simulink model "mfordmodel_v1"  (R2023a)
settings: Solver=ode45  StartTime=0.0  StopTime=10.0  RelTol=1e-3  EnableMultiTasking=on
undefined symbols (not defined in the file): ABV_RATIO_SW, AC_OFF_DLY, ACLOD, AUTO_TRNS_SW, BRAKE_DNDT_X, BZZRPM, BZZRPM_ALT, BZZTM, BZZTM_ALT, CMD_LITOFF, CMD_STABLE, CO_ST_ECT__A, COOL_BASE, DAS_BKDLY_A, DAS_CNT, DAS_CTDLY, DAS_LC_SW__A, DASCLP_5INH, DASCTL, DASMHYST, DASMPH, DEBYCP, DES_BASE, DPNEU_MUL, DSDRPM_DN_TC, DSDRPM_OFF, DSDRPM_UP_TC, EDF_DELAY, EDFHP, ETC_CL_TP, ETC_HP, GR_CM_CREEP, HCAM_ACT_CLP, HEDFHP, HEDFRPM, HICAM_PS, IAC_CAL_SW, IAC_ER_TM1, IAC_ER_TM2, IAC_ER_TM4, IAC_HI_LIM__A, IAC_ISFL_OBD, IAC_KAM_SW, IAC_LO_LIM__A, IAC_MON_TM, IAC_OT_REQ, IAC_RUN_TM, IAC_TP_OBD, IAC_TR_DAS, IAC_TST_DC, ID_DAS__A, ID_NOVS__A, IDVS_CH__A, IDVS_SL__A, IPSI_SW, IPSIDLY, IS_DRBASE__A, IS_DRBASE_A__A, IS_NUBASE__A, IS_NUBASE_A__A ... (+35)
libraries: simulink x2
(part 1 of 12)
settings Model: ModifiedHistory=Current Utils Library:utils53_v1.mdl  ExtModeTrigMode=oneshot  Creator=myunt  LastModifiedBy=dkar
settings SolverCC: AlgebraicLoopSolver=TrustRegion
settings DataIOCC: SaveFormat=Array  SignalLoggingSaveFormat=ModelDataLogs  ReturnWorkspaceOutputs=off
settings OptimizationCC: BooleanDataType=off  ExpressionDepthLimit=2147483647  InitFltsAndDblsToZero=on  EfficientMapNaN2IntZero=off  LifeSpan=inf
settings DebuggingCC: SaveWithParameterizedLinksMsg=none  UnderspecifiedInitializationDetection=Classic  MergeDetectMultiDrivingBlocksExec=none  CheckExecutionContextPreStartOutputMsg=on  SignalResolutionControl=TryResolveAllWithWarning  MultiTaskDSMMsg=warning  MultiTaskCondExecSysMsg=none  FcnCallInpInsideContextMsg=warning  UnconnectedInputMsg=warning  UnconnectedOutputMsg=warning  UnconnectedLineMsg=warning  StateNameClashWarn=warning  SFUnexpectedBacktrackingDiag=warning  SFNoUnconditionalDefaultTransitionDiag=warning  SFExecutionAtInitializationDiag=none  ArithmeticOperatorsInVariantConditions=warning
settings HardwareCC: ProdBitPerPointer=32  ProdBitPerSizeT=32  ProdBitPerPtrDiffT=32  ProdLargestAtomicFloat=None  ProdIntDivRoundTo=Undefined  ProdEndianess=Unspecified  ProdWordSize=32  ProdHWDeviceType=32-bit Generic  TargetUnknown=on
settings ModelReferenceCC: PropagateSignalLabelsOutOfModel=off
settings SFSimCC: SimUseLocalCustomCode=off  SimParseCustomCode=off  CustomCodeUndefinedFunction=UseInterfaceOnly
settings RTWCC: RTWUseLocalCustomCode=off
settings CodeAppCC: StateflowObjectComments=on
settings GRTTargetCC: TargetFcnLib=ansi_tfl_tmw.mat  TargetLangStandard=C89/C90 (ANSI)  CombineOutputUpdateFcns=off  GRTInterface=on
settings ConfigComp: CovMetricSettings=dw  CovSaveCumulativeToWorkspaceVar=on  CovSaveSingleToWorkspaceVar=on

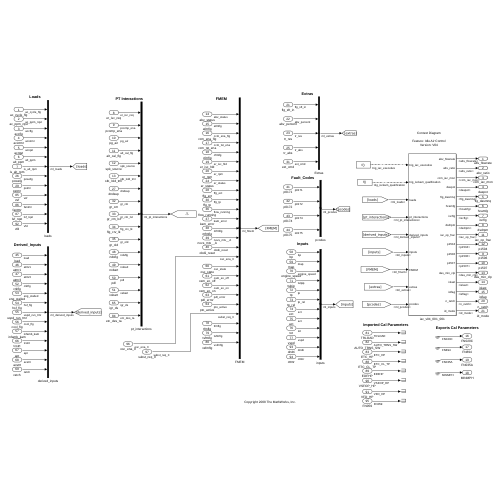
[thumbnail: Simulink's stored preview of the top-level diagram]
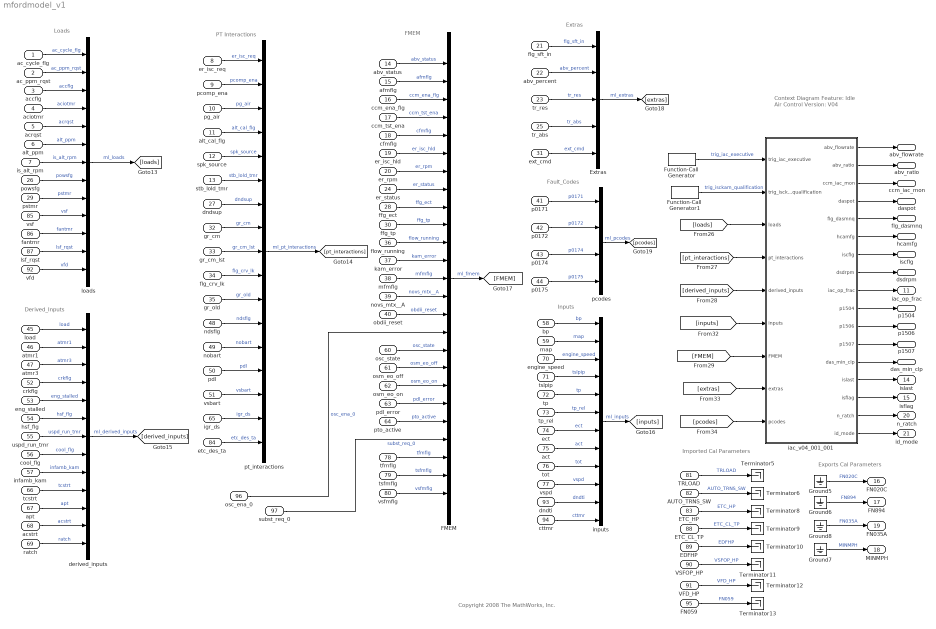
== system mfordmodel_v1 ==
  note: Loads
  note: PT Interactions
  note: Derived_Inputs
  note: Inputs
  note: FMEM
  note: Extras
  note: Context Diagram
      |
      | Feature: Idle Air Control
      | Version: V04
  note: Imported Cal Parameters
  note: Exports Cal Parameters
  note: Fault_Codes
  note: Copyright 2008 The MathWorks, Inc.
  ac_cycle_flg : Inport
  ac_ppm_rqst : Inport  Port=2
  accflg : Inport  Port=3
  aciotmr : Inport  Port=4
  acrqst : Inport  Port=5
  alt_ppm : Inport  Port=6
  is_alt_rpm : Inport  Port=7
  er_isc_req : Inport  Port=8
  pcomp_ena : Inport  Port=9
  pg_air : Inport  Port=10
  alt_cal_flg : Inport  Port=11
  spk_source : Inport  Port=12
  stb_lold_tmr : Inport  Port=13
  abv_status : Inport  Port=14
  afmflg : Inport  Port=15
  ccm_ena_flg : Inport  Port=16
  ccm_tst_ena : Inport  Port=17
  cfmflg : Inport  Port=18
  er_isc_hld : Inport  Port=19
  er_rpm : Inport  Port=20
  flg_sft_in : Inport  Port=21
  abv_percent : Inport  Port=22
  tr_res : Inport  Port=23
  er_status : Inport  Port=24
  tr_abs : Inport  Port=25
  powsfg : Inport  Port=26
  dndsup : Inport  Port=27
  ffg_ect : Inport  Port=28
  pstmr : Inport  Port=29
  ffg_tp : Inport  Port=30
  ext_cmd : Inport  Port=31
  gr_cm : Inport  Port=32
  gr_cm_lst : Inport  Port=33
  flg_crv_lk : Inport  Port=34
  gr_old : Inport  Port=35
  flow_running : Inport  Port=36
  kam_error : Inport  Port=37
  mfmflg : Inport  Port=38
  novs_mtx__A : Inport  Port=39
  obdii_reset : Inport  Port=40
  p0171 : Inport  Port=41
  p0172 : Inport  Port=42
  p0174 : Inport  Port=43
  p0175 : Inport  Port=44
  load : Inport  Port=45
  atmr1 : Inport  Port=46
  atmr3 : Inport  Port=47
  ndsflg : Inport  Port=48
  nobart : Inport  Port=49
  pdl : Inport  Port=50
  vsbart : Inport  Port=51
  crkflg : Inport  Port=52
  eng_stalled : Inport  Port=53
  hsf_flg : Inport  Port=54
  uspd_run_tmr : Inport  Port=55
  cool_flg : Inport  Port=56
  infamb_kam : Inport  Port=57
  bp : Inport  Port=58
  map : Inport  Port=59
  osc_state : Inport  Port=60
  osm_eo_off : Inport  Port=61
  osm_eo_on : Inport  Port=62
  pdl_error : Inport  Port=63
  pto_active : Inport  Port=64
  igr_ds : Inport  Port=65
  tcstrt : Inport  Port=66
  apt : Inport  Port=67
  acstrt : Inport  Port=68
  ratch : Inport  Port=69
  engine_speed : Inport  Port=70
  tslpip : Inport  Port=71
  tp : Inport  Port=72
  tp_rel : Inport  Port=73
  ect : Inport  Port=74
  act : Inport  Port=75
  tot : Inport  Port=76
  vspd : Inport  Port=77
  tfmflg : Inport  Port=78
  tsfmflg : Inport  Port=79
  vsfmflg : Inport  Port=80
  TRLOAD : Inport  Port=81
  AUTO_TRNS_SW : Inport  Port=82
  ETC_HP : Inport  Port=83
  etc_des_ta : Inport  Port=84
  vsf : Inport  Port=85
  fantmr : Inport  Port=86
  lsf_rqst : Inport  Port=87
  ETC_CL_TP : Inport  Port=88
  EDFHP : Inport  Port=89
  VSFOP_HP : Inport  Port=90
  VFD_HP : Inport  Port=91
  vfd : Inport  Port=92
  dndti : Inport  Port=93
  cttmr : Inport  Port=94
  FN059 : Inport  Port=95
  osc_ena_0 : Inport  Port=96
  subst_req_0 : Inport  Port=97
  Extras : Mux  Inputs=5
  FMEM : Mux  Inputs=25
  Function-Call Generator : simulink/Ports & Subsystems/Function-Call Generator  sample_time=0.1  numberOfIterations=1  DisallowWideOutput=off
  Function-Call Generator1 : simulink/Ports & Subsystems/Function-Call Generator  sample_time=0.030  numberOfIterations=1  DisallowWideOutput=off
  Ground{5..8} (4 alike) : Ground
  Terminator{5..6,8..13} (8 alike) : Terminator
  derived_inputs : Mux  Inputs=13
  iac_v04_001_001 : Subsystem
  inputs : Mux  Inputs=12
  loads : Mux  Inputs=13
  pcodes : Mux  Inputs=p0171,p0172,p0174,p0175
  pt_interactions : Mux  Inputs=17
  abv_flowrate : Outport
  abv_ratio : Outport  Port=2
  ccm_iac_mon : Outport  Port=3
  daspot : Outport  Port=4
  flg_dasmnq : Outport  Port=5
  hcamfg : Outport  Port=6
  iscflg : Outport  Port=7
  dsdrpm : Outport  Port=8
  p1506 : Outport  Port=9
  p1507 : Outport  Port=10
  iac_op_frac : Outport  Port=11
  p1504 : Outport  Port=12
  das_min_clp : Outport  Port=13
  islast : Outport  Port=14
  isflag : Outport  Port=15
  FN020C : Outport  Port=16
  FN894 : Outport  Port=17
  MINMPH : Outport  Port=18
  FN035A : Outport  Port=19
  n_ratch : Outport  Port=20
  id_mode : Outport  Port=21
  wires:
  ac_ppm_rqst/1 -> loads/2  "ac_ppm_rqst"
  ac_cycle_flg/1 -> loads/1  "ac_cycle_flg"
  loads/1 -> [loads]  "ml_loads"
  er_isc_req/1 -> pt_interactions/1  "er_isc_req"
  pg_air/1 -> pt_interactions/3  "pg_air"
  pcomp_ena/1 -> pt_interactions/2  "pcomp_ena"
  spk_source/1 -> pt_interactions/5  "spk_source"
  stb_lold_tmr/1 -> pt_interactions/6  "stb_lold_tmr"
  alt_cal_flg/1 -> pt_interactions/4  "alt_cal_flg"
  pt_interactions/1 -> [pt_interactions]  "ml_pt_interactions"
  Extras/1 -> [extras]  "ml_extras"
  accflg/1 -> loads/3  "accflg"
  aciotmr/1 -> loads/4  "aciotmr"
  acrqst/1 -> loads/5  "acrqst"
  is_alt_rpm/1 -> loads/7  "is_alt_rpm"
  alt_ppm/1 -> loads/6  "alt_ppm"
  [pt_interactions] -> iac_v04_001_001/4(pt_interactions)
  [derived_inputs] -> iac_v04_001_001/5(derived_inputs)
  [inputs] -> iac_v04_001_001/6(inputs)
  [extras] -> iac_v04_001_001/8(extras)
  TRLOAD/1 -> Terminator5/1  "TRLOAD"
  AUTO_TRNS_SW/1 -> Terminator6/1  "AUTO_TRNS_SW"
  Ground5/1 -> FN020C/1  "FN020C"
  Ground6/1 -> FN894/1  "FN894"
  [pcodes] -> iac_v04_001_001/9(pcodes)
  Ground7/1 -> MINMPH/1  "MINMPH"
  Ground8/1 -> FN035A/1  "FN035A"
  FMEM/1 -> [FMEM]  "ml_fmem"
  osc_state/1 -> FMEM/17  "osc_state"
  osm_eo_off/1 -> FMEM/18  "osm_eo_off"
  osm_eo_on/1 -> FMEM/19  "osm_eo_on"
  pdl_error/1 -> FMEM/20  "pdl_error"
  pto_active/1 -> FMEM/21  "pto_active"
  tfmflg/1 -> FMEM/23  "tfmflg"
  tsfmflg/1 -> FMEM/24  "tsfmflg"
  derived_inputs/1 -> [derived_inputs]  "ml_derived_inputs"
  load/1 -> derived_inputs/1  "load"
  atmr1/1 -> derived_inputs/2  "atmr1"
  atmr3/1 -> derived_inputs/3  "atmr3"
  crkflg/1 -> derived_inputs/4  "crkflg"
  eng_stalled/1 -> derived_inputs/5  "eng_stalled"
  hsf_flg/1 -> derived_inputs/6  "hsf_flg"
  uspd_run_tmr/1 -> derived_inputs/7  "uspd_run_tmr"
  cool_flg/1 -> derived_inputs/8  "cool_flg"
  infamb_kam/1 -> derived_inputs/9  "infamb_kam"
  tcstrt/1 -> derived_inputs/10  "tcstrt"
  apt/1 -> derived_inputs/11  "apt"
  acstrt/1 -> derived_inputs/12  "acstrt"
  ratch/1 -> derived_inputs/13  "ratch"
  osc_ena_0/1 -> FMEM/16  "osc_ena_0"
  subst_req_0/1 -> FMEM/22  "subst_req_0"
  dndsup/1 -> pt_interactions/7  "dndsup"
  gr_cm/1 -> pt_interactions/8  "gr_cm"
  gr_cm_lst/1 -> pt_interactions/9  "gr_cm_lst"
  flg_crv_lk/1 -> pt_interactions/10  "flg_crv_lk"
  gr_old/1 -> pt_interactions/11  "gr_old"
  ndsflg/1 -> pt_interactions/12  "ndsflg"
  pdl/1 -> pt_interactions/14  "pdl"
  vsbart/1 -> pt_interactions/15  "vsbart"
  igr_ds/1 -> pt_interactions/16  "igr_ds"
  etc_des_ta/1 -> pt_interactions/17  "etc_des_ta"
  nobart/1 -> pt_interactions/13  "nobart"
  powsfg/1 -> loads/8  "powsfg"
  pstmr/1 -> loads/9  "pstmr"
  vsf/1 -> loads/10  "vsf"
  fantmr/1 -> loads/11  "fantmr"
  lsf_rqst/1 -> loads/12  "lsf_rqst"
  vfd/1 -> loads/13  "vfd"
  vsfmflg/1 -> FMEM/25  "vsfmflg"
  abv_status/1 -> FMEM/1  "abv_status"
  afmflg/1 -> FMEM/2  "afmflg"
  ccm_ena_flg/1 -> FMEM/3  "ccm_ena_flg"
  ccm_tst_ena/1 -> FMEM/4  "ccm_tst_ena"
  cfmflg/1 -> FMEM/5  "cfmflg"
  er_isc_hld/1 -> FMEM/6  "er_isc_hld"
  er_status/1 -> FMEM/8  "er_status"
  ffg_ect/1 -> FMEM/9  "ffg_ect"
  ffg_tp/1 -> FMEM/10  "ffg_tp"
  flow_running/1 -> FMEM/11  "flow_running"
  er_rpm/1 -> FMEM/7  "er_rpm"
  kam_error/1 -> FMEM/12  "kam_error"
  mfmflg/1 -> FMEM/13  "mfmflg"
  novs_mtx__A/1 -> FMEM/14  "novs_mtx__A"
  obdii_reset/1 -> FMEM/15  "obdii_reset"
  flg_sft_in/1 -> Extras/1  "flg_sft_in"
  abv_percent/1 -> Extras/2  "abv_percent"
  tr_res/1 -> Extras/3  "tr_res"
  tr_abs/1 -> Extras/4  "tr_abs"
  ext_cmd/1 -> Extras/5  "ext_cmd"
  pcodes/1 -> [pcodes]  "ml_pcodes"
  p0171/1 -> pcodes/1  "p0171"
  p0172/1 -> pcodes/2  "p0172"
  p0174/1 -> pcodes/3  "p0174"
  p0175/1 -> pcodes/4  "p0175"
  ect/1 -> inputs/7  "ect"
  act/1 -> inputs/8  "act"
  tot/1 -> inputs/9  "tot"
  tp/1 -> inputs/5  "tp"
  tp_rel/1 -> inputs/6  "tp_rel"
  tslpip/1 -> inputs/4  "tslpip"
  engine_speed/1 -> inputs/3  "engine_speed"
  map/1 -> inputs/2  "map"
  bp/1 -> inputs/1  "bp"
  vspd/1 -> inputs/10  "vspd"
  inputs/1 -> [inputs]  "ml_inputs"
  dndti/1 -> inputs/11  "dndti"
  cttmr/1 -> inputs/12  "cttmr"
  ETC_HP/1 -> Terminator8/1  "ETC_HP"
  ETC_CL_TP/1 -> Terminator9/1  "ETC_CL_TP"
  EDFHP/1 -> Terminator10/1  "EDFHP"
  VSFOP_HP/1 -> Terminator11/1  "VSFOP_HP"
  VFD_HP/1 -> Terminator12/1  "VFD_HP"
  iac_v04_001_001/3(ccm_iac_mon) -> ccm_iac_mon/1
  iac_v04_001_001/5(flg_dasmnq) -> flg_dasmnq/1
  iac_v04_001_001/12(p1507) -> p1507/1
  iac_v04_001_001/2(abv_ratio) -> abv_ratio/1
  iac_v04_001_001/4(daspot) -> daspot/1
  iac_v04_001_001/6(hcamfg) -> hcamfg/1
  iac_v04_001_001/7(iscflg) -> iscflg/1
  iac_v04_001_001/11(p1506) -> p1506/1
  iac_v04_001_001/1(abv_flowrate) -> abv_flowrate/1
  iac_v04_001_001/8(dsdrpm) -> dsdrpm/1
  iac_v04_001_001/9(iac_op_frac) -> iac_op_frac/1
  iac_v04_001_001/10(p1504) -> p1504/1
  iac_v04_001_001/13(das_min_clp) -> das_min_clp/1
  iac_v04_001_001/14(islast) -> islast/1
  iac_v04_001_001/15(isflag) -> isflag/1
  iac_v04_001_001/16(n_ratch) -> n_ratch/1
  iac_v04_001_001/17(id_mode) -> id_mode/1
  [loads] -> iac_v04_001_001/3(loads)
  [FMEM] -> iac_v04_001_001/7(FMEM)
  Function-Call Generator1/1 -> iac_v04_001_001/2(trig_isckam_qualification)  "trig_isckam_qualification"
  Function-Call Generator/1 -> iac_v04_001_001/1(trig_iac_executive)  "trig_iac_executive"
  FN059/1 -> Terminator13/1  "FN059"

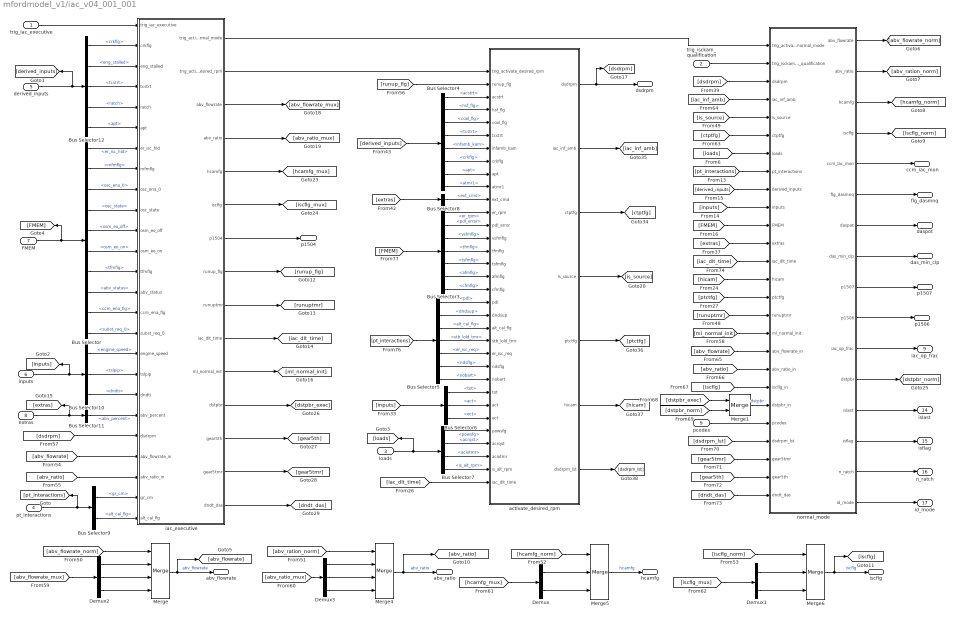
== system mfordmodel_v1/iac_v04_001_001 ==
  trig_iac_executive : Inport
  trig_isckam_qualification : Inport  Port=2
  loads : Inport  Port=3
  pt_interactions : Inport  Port=4
  derived_inputs : Inport  Port=5
  inputs : Inport  Port=6
  FMEM : Inport  Port=7
  extras : Inport  Port=8
  pcodes : Inport  Port=9
  Bus Selector : BusSelector  OutputSignals=er_isc_hld,mfmflg,osc_ena_0,osc_state,osm_eo_off,osm_eo_on,tfmflg,abv_status,ccm_ena_flg,subst_req_0
  Bus Selector10 : BusSelector  OutputSignals=engine_speed,tslpip,dndti
  Bus Selector11 : BusSelector  OutputSignals=abv_percent
  Bus Selector12 : BusSelector  OutputSignals=crkflg,eng_stalled,tcstrt,ratch,apt
  Bus Selector3 : BusSelector  OutputSignals=er_rpm,pdl_error,vsfmflg,tfmflg,tsfmflg,afmflg,cfmflg
  Bus Selector4 : BusSelector  OutputSignals=acstrt,hsf_flg,cool_flg,tcstrt,infamb_kam,crkflg,apt,atmr1
  Bus Selector5 : BusSelector  OutputSignals=pdl,dndsup,alt_cal_flg,stb_lold_tmr,er_isc_req,ndsflg,nobart
  Bus Selector6 : BusSelector  OutputSignals=tot,act,ect
  Bus Selector7 : BusSelector  OutputSignals=powsfg,acrqst,aciotmr,is_alt_rpm
  Bus Selector8 : BusSelector  OutputSignals=ext_cmd
  Bus Selector9 : BusSelector  OutputSignals=gr_cm,alt_cal_flg
  Demux : Demux  Outputs=2
      settings: DisplayOption=none
  Demux1 : Demux  Outputs=2
      settings: DisplayOption=none
  Demux2 : Demux  Outputs=3
      settings: DisplayOption=none
  Demux3 : Demux  Outputs=3
      settings: DisplayOption=none
  Merge : Merge  Inputs=4
  Merge1 : Merge
  Merge4 : Merge  Inputs=4
  Merge5 : Merge  Inputs=3
  Merge6 : Merge  Inputs=3
  activate_desired_rpm : Subsystem
  iac_executive : Subsystem
  normal_mode : Subsystem
  abv_flowrate : Outport
  abv_ratio : Outport  Port=2
  ccm_iac_mon : Outport  Port=3
  daspot : Outport  Port=4
  flg_dasmnq : Outport  Port=5
  hcamfg : Outport  Port=6
  iscflg : Outport  Port=7
  dsdrpm : Outport  Port=8
  iac_op_frac : Outport  Port=9
  p1504 : Outport  Port=10
  p1506 : Outport  Port=11
  p1507 : Outport  Port=12
  das_min_clp : Outport  Port=13
  islast : Outport  Port=14
  isflag : Outport  Port=15
  n_ratch : Outport  Port=16
  id_mode : Outport  Port=17
  wires:
  normal_mode/16(id_mode) -> id_mode/1
  normal_mode/15(n_ratch) -> n_ratch/1
  normal_mode/11(iac_op_frac) -> iac_op_frac/1
  normal_mode/9(p1507) -> p1507/1
  normal_mode/6(flg_dasmnq) -> flg_dasmnq/1
  normal_mode/5(ccm_iac_mon) -> ccm_iac_mon/1
  normal_mode/7(daspot) -> daspot/1
  normal_mode/8(das_min_clp) -> das_min_clp/1
  normal_mode/14(isflag) -> isflag/1
  normal_mode/13(islast) -> islast/1
  normal_mode/10(p1506) -> p1506/1
  Demux1/1 -> Merge6/2
  Demux1/2 -> Merge6/3
  Merge6/1 -> iscflg/1, [iscflg]  "iscflg"
  [iscflg_mux] -> Demux1/1
  [iscflg_norm] -> Merge6/1
  Demux/1 -> Merge5/2
  Demux/2 -> Merge5/3
  Merge5/1 -> hcamfg/1  "hcamfg"
  [hcamfg_mux] -> Demux/1
  Demux2/3 -> Merge/4
  Demux2/1 -> Merge/2
  [abv_flowrate_norm] -> Merge/1
  Merge/1 -> abv_flowrate/1, [abv_flowrate]  "abv_flowrate"
  [abv_flowrate_mux] -> Demux2/1
  Demux2/2 -> Merge/3
  derived_inputs/1 -> Bus Selector12/1, [derived_inputs]
  Bus Selector12/5 -> iac_executive/6(apt)  "<apt>"
  pt_interactions/1 -> Bus Selector9/1, [pt_interactions]
  Bus Selector9/1 -> iac_executive/24(gr_cm)  "<gr_cm>"
  Bus Selector9/2 -> iac_executive/25(alt_cal_flg)  "<alt_cal_flg>"
  extras/1 -> Bus Selector11/1, [extras]
  Bus Selector11/1 -> iac_executive/20(abv_percent)  "<abv_percent>"
  [dsdrpm] -> iac_executive/21(dsdrpm)
  [abv_flowrate] -> iac_executive/22(abv_flowrate_in)
  [abv_ratio] -> iac_executive/23(abv_ratio_in)
  inputs/1 -> Bus Selector10/1, [inputs]
  Bus Selector10/3 -> iac_executive/19(dndti)  "<dndti>"
  Bus Selector10/1 -> iac_executive/17(engine_speed)  "<engine_speed>"
  Bus Selector10/2 -> iac_executive/18(tslpip)  "<tslpip>"
  FMEM/1 -> Bus Selector/1, [FMEM]
  Bus Selector/2 -> iac_executive/8(mfmflg)  "<mfmflg>"
  Bus Selector/3 -> iac_executive/9(osc_ena_0)  "<osc_ena_0>"
  Bus Selector/4 -> iac_executive/10(osc_state)  "<osc_state>"
  Bus Selector/5 -> iac_executive/11(osm_eo_off)  "<osm_eo_off>"
  Bus Selector/6 -> iac_executive/12(osm_eo_on)  "<osm_eo_on>"
  Bus Selector/7 -> iac_executive/13(tfmflg)  "<tfmflg>"
  Bus Selector/8 -> iac_executive/14(abv_status)  "<abv_status>"
  Bus Selector/10 -> iac_executive/16(subst_req_0)  "<subst_req_0>"
  Bus Selector/9 -> iac_executive/15(ccm_ena_flg)  "<ccm_ena_flg>"
  Bus Selector12/1 -> iac_executive/2(crkflg)  "<crkflg>"
  Bus Selector12/2 -> iac_executive/3(eng_stalled)  "<eng_stalled>"
  trig_iac_executive/1 -> iac_executive/1(trig_iac_executive)
  Bus Selector/1 -> iac_executive/7(er_isc_hld)  "<er_isc_hld>"
  Bus Selector12/3 -> iac_executive/4(tcstrt)  "<tcstrt>"
  Bus Selector12/4 -> iac_executive/5(ratch)  "<ratch>"
  iac_executive/7(p1504) -> p1504/1
  Bus Selector5/7 -> activate_desired_rpm/25(nobart)  "<nobart>"
  [dstpbr_exec] -> Merge1/1
  [dstpbr_norm] -> Merge1/2
  [gear5tmr] -> normal_mode/24(gear5tmr)
  [dndt_das] -> normal_mode/26(dndt_das)
  [gear5th] -> normal_mode/25(gear5th)
  pcodes/1 -> normal_mode/22(pcodes)
  iac_executive/15(dndt_das) -> [dndt_das]
  iac_executive/14(gear5tmr) -> [gear5tmr]
  iac_executive/13(gear5th) -> [gear5th]
  [derived_inputs] -> Bus Selector4/1
  Bus Selector8/1 -> activate_desired_rpm/11(ext_cmd)  "<ext_cmd>"
  [extras] -> Bus Selector8/1
  [FMEM] -> Bus Selector3/1
  Bus Selector3/1 -> activate_desired_rpm/12(er_rpm)  "<er_rpm>"
  Bus Selector3/2 -> activate_desired_rpm/13(pdl_error)  "<pdl_error>"
  Bus Selector3/3 -> activate_desired_rpm/14(vsfmflg)  "<vsfmflg>"
  Bus Selector3/4 -> activate_desired_rpm/15(tfmflg)  "<tfmflg>"
  Bus Selector3/5 -> activate_desired_rpm/16(tsfmflg)  "<tsfmflg>"
  Bus Selector3/6 -> activate_desired_rpm/17(afmflg)  "<afmflg>"
  Bus Selector3/7 -> activate_desired_rpm/18(cfmflg)  "<cfmflg>"
  [pt_interactions] -> Bus Selector5/1
  [dsdrpm_lst] -> normal_mode/23(dsdrpm_lst)
  [FMEM] -> normal_mode/11(FMEM)
  [inputs] -> normal_mode/10(inputs)
  [dsdrpm] -> normal_mode/3(dsdrpm)
  [hicam] -> normal_mode/14(hicam)
  [ptctfg] -> normal_mode/15(ptctfg)
  trig_isckam_qualification/1 -> normal_mode/2(trig_isckam_qualification)
  activate_desired_rpm/7(dsdrpm_lst) -> [dsdrpm_lst]
  normal_mode/1(abv_flowrate) -> [abv_flowrate_norm]
  normal_mode/3(hcamfg) -> [hcamfg_norm]
  normal_mode/4(iscflg) -> [iscflg_norm]
  normal_mode/2(abv_ratio) -> [abv_ration_norm]
  Bus Selector7/1 -> activate_desired_rpm/29(powsfg)  "<powsfg>"
  Bus Selector7/2 -> activate_desired_rpm/30(acrqst)  "<acrqst>"
  Bus Selector7/3 -> activate_desired_rpm/31(aciotmr)  "<aciotmr>"
  Bus Selector7/4 -> activate_desired_rpm/32(is_alt_rpm)  "<is_alt_rpm>"
  Bus Selector4/1 -> activate_desired_rpm/3(acstrt)  "<acstrt>"
  Bus Selector4/2 -> activate_desired_rpm/4(hsf_flg)  "<hsf_flg>"
  Bus Selector4/3 -> activate_desired_rpm/5(cool_flg)  "<cool_flg>"
  Bus Selector4/4 -> activate_desired_rpm/6(tcstrt)  "<tcstrt>"
  Bus Selector4/5 -> activate_desired_rpm/7(infamb_kam)  "<infamb_kam>"
  Bus Selector4/6 -> activate_desired_rpm/8(crkflg)  "<crkflg>"
  Bus Selector4/7 -> activate_desired_rpm/9(apt)  "<apt>"
  Bus Selector4/8 -> activate_desired_rpm/10(atmr1)  "<atmr1>"
  Bus Selector5/1 -> activate_desired_rpm/19(pdl)  "<pdl>"
  Bus Selector5/2 -> activate_desired_rpm/20(dndsup)  "<dndsup>"
  Bus Selector5/3 -> activate_desired_rpm/21(alt_cal_flg)  "<alt_cal_flg>"
  Bus Selector5/4 -> activate_desired_rpm/22(stb_lold_tmr)  "<stb_lold_tmr>"
  Bus Selector5/5 -> activate_desired_rpm/23(er_isc_req)  "<er_isc_req>"
  Bus Selector5/6 -> activate_desired_rpm/24(ndsflg)  "<ndsflg>"
  [runup_flg] -> activate_desired_rpm/2(runup_flg)
  activate_desired_rpm/2(iac_inf_amb) -> [iac_inf_amb]
  activate_desired_rpm/3(ctptfg) -> [ctptfg]
  activate_desired_rpm/4(is_source) -> [is_source]
  activate_desired_rpm/5(ptctfg) -> [ptctfg]
  [iac_dlt_time] -> activate_desired_rpm/33(iac_dlt_time)
  activate_desired_rpm/6(hicam) -> [hicam]
  Merge1/1 -> normal_mode/21(dstpbr_in)  "dstpbr"
  loads/1 -> Bus Selector7/1, [loads]
  Bus Selector6/1 -> activate_desired_rpm/26(tot)  "<tot>"
  Bus Selector6/2 -> activate_desired_rpm/27(act)  "<act>"
  Bus Selector6/3 -> activate_desired_rpm/28(ect)  "<ect>"
  [inputs] -> Bus Selector6/1
  [hcamfg_norm] -> Merge5/1
  activate_desired_rpm/1(dsdrpm) -> [dsdrpm], dsdrpm/1
  iac_executive/1(trig_activate_normal_mode) -> normal_mode/1(trig_activate_normal_mode)
  iac_executive/8(runup_flg) -> [runup_flg]
  iac_executive/10(iac_dlt_time) -> [iac_dlt_time]
  iac_executive/9(runuptmr) -> [runuptmr]
  iac_executive/2(trig_activate_desired_rpm) -> activate_desired_rpm/1(trig_activate_desired_rpm)
  iac_executive/11(ml_normal_init) -> [ml_normal_init]
  iac_executive/3(abv_flowrate) -> [abv_flowrate_mux]
  iac_executive/4(abv_ratio) -> [abv_ratio_mux]
  iac_executive/5(hcamfg) -> [hcamfg_mux]
  iac_executive/6(iscflg) -> [iscflg_mux]
  iac_executive/12(dstpbr) -> [dstpbr_exec]
  Demux3/3 -> Merge4/4
  [abv_ration_norm] -> Merge4/1
  Demux3/1 -> Merge4/2
  Demux3/2 -> Merge4/3
  Merge4/1 -> abv_ratio/1, [abv_ratio]  "abv_ratio"
  [abv_ratio_mux] -> Demux3/1
  [loads] -> normal_mode/7(loads)
  [pt_interactions] -> normal_mode/8(pt_interactions)
  [derived_inputs] -> normal_mode/9(derived_inputs)
  [extras] -> normal_mode/12(extras)
  [iac_dlt_time] -> normal_mode/13(iac_dlt_time)
  [is_source] -> normal_mode/5(is_source)
  [ctptfg] -> normal_mode/6(ctptfg)
  [iac_inf_amb] -> normal_mode/4(iac_inf_amb)
  [runuptmr] -> normal_mode/16(runuptmr)
  [ml_normal_init] -> normal_mode/17(ml_normal_init)
  [abv_flowrate] -> normal_mode/18(abv_flowrate_in)
  [abv_ratio] -> normal_mode/19(abv_ratio_in)
  [iscflg] -> normal_mode/20(iscflg_in)
  normal_mode/12(dstpbr) -> [dstpbr_norm]

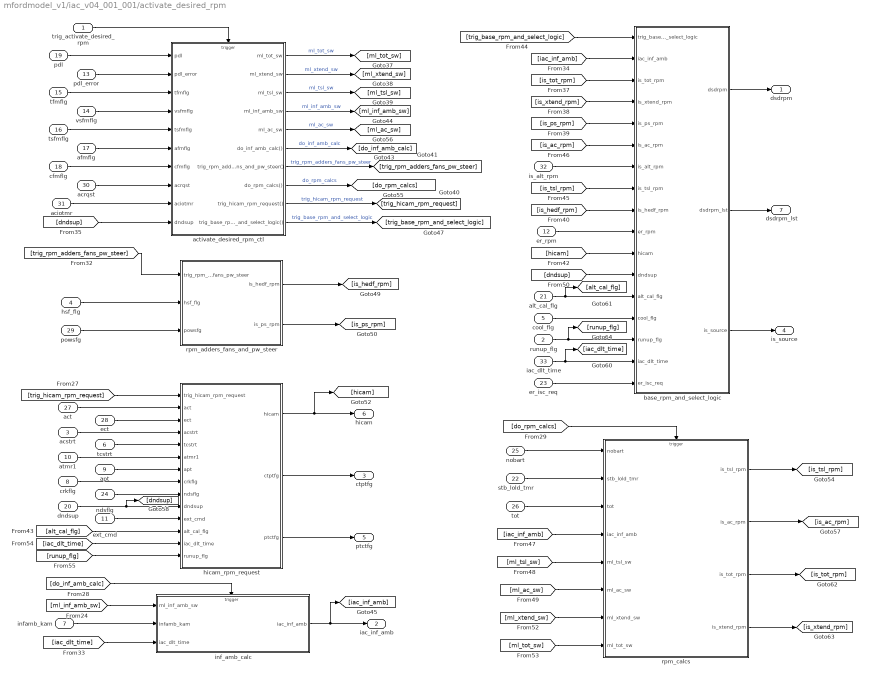
== system mfordmodel_v1/iac_v04_001_001/activate_desired_rpm ==
  trig_activate_desired_rpm : Inport
  runup_flg : Inport  Port=2
  acstrt : Inport  Port=3
  hsf_flg : Inport  Port=4
  cool_flg : Inport  Port=5
  tcstrt : Inport  Port=6
  infamb_kam : Inport  Port=7
  crkflg : Inport  Port=8
  apt : Inport  Port=9
  atmr1 : Inport  Port=10
  ext_cmd : Inport  Port=11
  er_rpm : Inport  Port=12
  pdl_error : Inport  Port=13
  vsfmflg : Inport  Port=14
  tfmflg : Inport  Port=15
  tsfmflg : Inport  Port=16
  afmflg : Inport  Port=17
  cfmflg : Inport  Port=18
  pdl : Inport  Port=19
  dndsup : Inport  Port=20
  alt_cal_flg : Inport  Port=21
  stb_lold_tmr : Inport  Port=22
  er_isc_req : Inport  Port=23
  ndsflg : Inport  Port=24
  nobart : Inport  Port=25
  tot : Inport  Port=26
  act : Inport  Port=27
  ect : Inport  Port=28
  powsfg : Inport  Port=29
  acrqst : Inport  Port=30
  aciotmr : Inport  Port=31
  is_alt_rpm : Inport  Port=32
  iac_dlt_time : Inport  Port=33
  activate_desired_rpm_ctl : Stateflow chart  TreatAsAtomicUnit=on
  base_rpm_and_select_logic : Subsystem
  hicam_rpm_request : Subsystem
  inf_amb_calc : Subsystem  TreatAsAtomicUnit=on  mask(inf_amb_calc){}
      mask help: TBD
      mask Display:
      | disp('
      | IF (ml_inf_amb_sw == 1)  THEN                              \n
      | iac_inf_amb = infamb_kam                              \n
      | ELSE IF (ml_inf_amb_sw == 2) THEN                     \n
      | iac_inf_amb = rolav_tc (iac_inf_amb,              \n
      | 254.0, iac_delta_time, 16)\n
      | ENDIF                                                                      ')
  rpm_adders_fans_and_pw_steer : Subsystem  mask(rpm_adders_fans_and_pw_steer){}
      mask help: Calculate the HEDF and PS RPM requests.
      mask Display:
      | disp('
      | IF ( ( HEDFHP == 1) AND      \n
      | ( HSF_FLG == 1))      \n
      | is_hedf_rpm = HEDFRPM\n
      | ELSE                                       \n
      | is_hedf_rpm = 0                \n
      | ENDIF                                    \n \n
      | IF (powsfg == 1)                     \n
      | is_ps_rpm = PS_RPM      \n
      | ELSE                                      \n
      | is_ps_rpm  = 0                  \n
      | ENDIF                                     ')
  rpm_calcs : Subsystem  TreatAsAtomicUnit=on  mask(rpm_calcs){}
      mask help: TBD
      mask Display:
      | disp('
      | IF (ml_tsl_sw == 1) THEN                          \n
      | is_tsl_rpm = 0.0                                    \n
      | ELSE IF (ml_tsl_sw == 2) THEN                \n
      | is_tsl_rpm = ( nobart * RT_CHAIN        \n
      |  * COAST_FRAC )\n
      | ENDIF                                                         \n\n
      | IF (ml_tot_sw == 1 ) THEN                         \n
      | is_tot_rpm = FN861R(tot)                   \n
      | ELSE IF (ml_tot_sw == 2) THEN                \n
      | is_tot_rpm = FN861(tot)                     \n
      | ENDIF                                                          \n\n
      | IF (ml_ac_sw == 1) THEN                           \n
      | is_ac_rpm = FNIAC_AC_N(iac_inf_amb)\n
      | ELSE IF (ml_ac_sw == 2) THEN                  \n
      | is_ac_rpm = FNIAC_AC_D(iac_inf_amb)\n
      | ELSE IF (ml_ac_sw == 3 THEN                   \n
      | is_ac_rpm = 0.0                                        \n
      | ENDIF                                                           \n\n
      | IF (is_xtend_rpm == 1) THEN                       \n
      | is_xtend_rpm = FN880N(stblold_tmr)     \n
      | ELSE IF (ml_xtend_sw == 2) THEN              \n
      | is_xtend_rpm = 0.0                                  \n
      | ENDIF                                                            ')
  dsdrpm : Outport
  iac_inf_amb : Outport  Port=2
  ctptfg : Outport  Port=3
  is_source : Outport  Port=4
  ptctfg : Outport  Port=5
  hicam : Outport  Port=6
  dsdrpm_lst : Outport  Port=7
  wires:
  vsfmflg/1 -> activate_desired_rpm_ctl/4(vsfmflg)
  alt_cal_flg/1 -> [alt_cal_flg], base_rpm_and_select_logic/13(alt_cal_flg)
  [ml_tot_sw] -> rpm_calcs/8(ml_tot_sw)
  [ml_xtend_sw] -> rpm_calcs/7(ml_xtend_sw)
  [ml_ac_sw] -> rpm_calcs/6(ml_ac_sw)
  [ml_tsl_sw] -> rpm_calcs/5(ml_tsl_sw)
  [iac_inf_amb] -> rpm_calcs/4(iac_inf_amb)
  tot/1 -> rpm_calcs/3(tot)
  stb_lold_tmr/1 -> rpm_calcs/2(stb_lold_tmr)
  nobart/1 -> rpm_calcs/1(nobart)
  rpm_calcs/4(is_xtend_rpm) -> [is_xtend_rpm]
  rpm_calcs/3(is_tot_rpm) -> [is_tot_rpm]
  rpm_calcs/2(is_ac_rpm) -> [is_ac_rpm]
  rpm_calcs/1(is_tsl_rpm) -> [is_tsl_rpm]
  [do_rpm_calcs] -> rpm_calcs/Trigger
  inf_amb_calc/1(iac_inf_amb) -> [iac_inf_amb], iac_inf_amb/1
  infamb_kam/1 -> inf_amb_calc/2(infamb_kam)
  [iac_dlt_time] -> inf_amb_calc/3(iac_dlt_time)
  [do_inf_amb_calc] -> inf_amb_calc/Trigger
  [ml_inf_amb_sw] -> inf_amb_calc/1(ml_inf_amb_sw)
  [trig_hicam_rpm_request] -> hicam_rpm_request/1(trig_hicam_rpm_request)
  act/1 -> hicam_rpm_request/2(act)
  ect/1 -> hicam_rpm_request/3(ect)
  acstrt/1 -> hicam_rpm_request/4(acstrt)
  tcstrt/1 -> hicam_rpm_request/5(tcstrt)
  atmr1/1 -> hicam_rpm_request/6(atmr1)
  apt/1 -> hicam_rpm_request/7(apt)
  crkflg/1 -> hicam_rpm_request/8(crkflg)
  ndsflg/1 -> hicam_rpm_request/9(ndsflg)
  dndsup/1 -> [dndsup], hicam_rpm_request/10(dndsup)
  ext_cmd/1 -> hicam_rpm_request/11(ext_cmd)
  [alt_cal_flg] -> hicam_rpm_request/12(alt_cal_flg)
  [iac_dlt_time] -> hicam_rpm_request/13(iac_dlt_time)
  [runup_flg] -> hicam_rpm_request/14(runup_flg)
  hicam_rpm_request/1(hicam) -> hicam/1, [hicam]
  hicam_rpm_request/2(ctptfg) -> ctptfg/1
  hicam_rpm_request/3(ptctfg) -> ptctfg/1
  rpm_adders_fans_and_pw_steer/2(is_ps_rpm) -> [is_ps_rpm]
  rpm_adders_fans_and_pw_steer/1(is_hedf_rpm) -> [is_hedf_rpm]
  powsfg/1 -> rpm_adders_fans_and_pw_steer/3(powsfg)
  hsf_flg/1 -> rpm_adders_fans_and_pw_steer/2(hsf_flg)
  [trig_rpm_adders_fans_pw_steer] -> rpm_adders_fans_and_pw_steer/1(trig_rpm_adders_fans_pw_steer)
  base_rpm_and_select_logic/2(dsdrpm_lst) -> dsdrpm_lst/1
  pdl/1 -> activate_desired_rpm_ctl/1(pdl)
  acrqst/1 -> activate_desired_rpm_ctl/8(acrqst)
  activate_desired_rpm_ctl/5(ml_ac_sw) -> [ml_ac_sw]  "ml_ac_sw"
  activate_desired_rpm_ctl/10(trig_base_rpm_and_select_logic()) -> [trig_base_rpm_and_select_logic]  "trig_base_rpm_and_select_logic"
  [dndsup] -> activate_desired_rpm_ctl/10(dndsup)
  pdl_error/1 -> activate_desired_rpm_ctl/2(pdl_error)
  activate_desired_rpm_ctl/4(ml_inf_amb_sw) -> [ml_inf_amb_sw]  "ml_inf_amb_sw"
  activate_desired_rpm_ctl/6(do_inf_amb_calc()) -> [do_inf_amb_calc]  "do_inf_amb_calc"
  activate_desired_rpm_ctl/7(trig_rpm_adders_fans_and_pw_steer()) -> [trig_rpm_adders_fans_pw_steer]  "trig_rpm_adders_fans_pw_steer"
  activate_desired_rpm_ctl/9(trig_hicam_rpm_request()) -> [trig_hicam_rpm_request]  "trig_hicam_rpm_request"
  activate_desired_rpm_ctl/3(ml_tsl_sw) -> [ml_tsl_sw]  "ml_tsl_sw"
  activate_desired_rpm_ctl/2(ml_xtend_sw) -> [ml_xtend_sw]  "ml_xtend_sw"
  activate_desired_rpm_ctl/1(ml_tot_sw) -> [ml_tot_sw]  "ml_tot_sw"
  trig_activate_desired_rpm/1 -> activate_desired_rpm_ctl/Trigger
  tfmflg/1 -> activate_desired_rpm_ctl/3(tfmflg)
  aciotmr/1 -> activate_desired_rpm_ctl/9(aciotmr)
  activate_desired_rpm_ctl/8(do_rpm_calcs()) -> [do_rpm_calcs]  "do_rpm_calcs"
  afmflg/1 -> activate_desired_rpm_ctl/6(afmflg)
  tsfmflg/1 -> activate_desired_rpm_ctl/5(tsfmflg)
  cfmflg/1 -> activate_desired_rpm_ctl/7(cfmflg)
  base_rpm_and_select_logic/3(is_source) -> is_source/1
  base_rpm_and_select_logic/1(dsdrpm) -> dsdrpm/1
  [trig_base_rpm_and_select_logic] -> base_rpm_and_select_logic/1(trig_base_rpm_and_select_logic)
  [hicam] -> base_rpm_and_select_logic/11(hicam)
  [iac_inf_amb] -> base_rpm_and_select_logic/2(iac_inf_amb)
  [dndsup] -> base_rpm_and_select_logic/12(dndsup)
  er_rpm/1 -> base_rpm_and_select_logic/10(er_rpm)
  [is_hedf_rpm] -> base_rpm_and_select_logic/9(is_hedf_rpm)
  [is_tsl_rpm] -> base_rpm_and_select_logic/8(is_tsl_rpm)
  is_alt_rpm/1 -> base_rpm_and_select_logic/7(is_alt_rpm)
  [is_ac_rpm] -> base_rpm_and_select_logic/6(is_ac_rpm)
  [is_ps_rpm] -> base_rpm_and_select_logic/5(is_ps_rpm)
  [is_xtend_rpm] -> base_rpm_and_select_logic/4(is_xtend_rpm)
  [is_tot_rpm] -> base_rpm_and_select_logic/3(is_tot_rpm)
  cool_flg/1 -> base_rpm_and_select_logic/14(cool_flg)
  er_isc_req/1 -> base_rpm_and_select_logic/17(er_isc_req)
  iac_dlt_time/1 -> [iac_dlt_time], base_rpm_and_select_logic/16(iac_dlt_time)
  runup_flg/1 -> base_rpm_and_select_logic/15(runup_flg), [runup_flg]

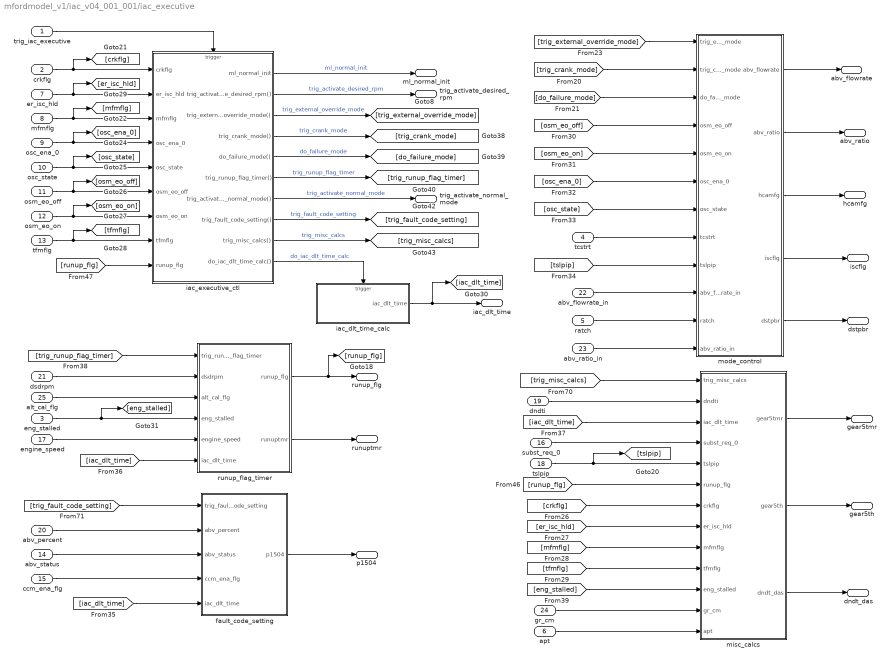
== system mfordmodel_v1/iac_v04_001_001/iac_executive ==
  trig_iac_executive : Inport
  crkflg : Inport  Port=2
  eng_stalled : Inport  Port=3
  tcstrt : Inport  Port=4
  ratch : Inport  Port=5
  apt : Inport  Port=6
  er_isc_hld : Inport  Port=7
  mfmflg : Inport  Port=8
  osc_ena_0 : Inport  Port=9
  osc_state : Inport  Port=10
  osm_eo_off : Inport  Port=11
  osm_eo_on : Inport  Port=12
  tfmflg : Inport  Port=13
  abv_status : Inport  Port=14
  ccm_ena_flg : Inport  Port=15
  subst_req_0 : Inport  Port=16
  engine_speed : Inport  Port=17
  tslpip : Inport  Port=18
  dndti : Inport  Port=19
  abv_percent : Inport  Port=20
  dsdrpm : Inport  Port=21
  abv_flowrate_in : Inport  Port=22
  abv_ratio_in : Inport  Port=23
  gr_cm : Inport  Port=24
  alt_cal_flg : Inport  Port=25
  fault_code_setting : Subsystem
  iac_dlt_time_calc : Subsystem  TreatAsAtomicUnit=on  mask(iac_dlt_time_calc){}
      mask help: Returns the elapse time (in seconds) since last called.
      mask Display:
      | fprintf('iac_dlt_time  = \n
      | clock - clock(previous) ')
  iac_executive_ctl : Stateflow chart  TreatAsAtomicUnit=on
  misc_calcs : Subsystem
  mode_control : Subsystem
  runup_flag_timer : Subsystem
  trig_activate_normal_mode : Outport
  trig_activate_desired_rpm : Outport  Port=2
  abv_flowrate : Outport  Port=3
  abv_ratio : Outport  Port=4
  hcamfg : Outport  Port=5
  iscflg : Outport  Port=6
  p1504 : Outport  Port=7
  runup_flg : Outport  Port=8
  runuptmr : Outport  Port=9
  iac_dlt_time : Outport  Port=10
  ml_normal_init : Outport  Port=11
  dstpbr : Outport  Port=12
  gear5th : Outport  Port=13
  gear5tmr : Outport  Port=14
  dndt_das : Outport  Port=15
  wires:
  apt/1 -> misc_calcs/13(apt)
  gr_cm/1 -> misc_calcs/12(gr_cm)
  [eng_stalled] -> misc_calcs/11(eng_stalled)
  eng_stalled/1 -> [eng_stalled], runup_flag_timer/4(eng_stalled)
  tslpip/1 -> [tslpip], misc_calcs/5(tslpip)
  [runup_flg] -> misc_calcs/6(runup_flg)
  [crkflg] -> misc_calcs/7(crkflg)
  [er_isc_hld] -> misc_calcs/8(er_isc_hld)
  [mfmflg] -> misc_calcs/9(mfmflg)
  [tfmflg] -> misc_calcs/10(tfmflg)
  subst_req_0/1 -> misc_calcs/4(subst_req_0)
  dndti/1 -> misc_calcs/2(dndti)
  [iac_dlt_time] -> misc_calcs/3(iac_dlt_time)
  [trig_misc_calcs] -> misc_calcs/1(trig_misc_calcs)
  misc_calcs/3(dndt_das) -> dndt_das/1
  misc_calcs/2(gear5th) -> gear5th/1
  misc_calcs/1(gear5tmr) -> gear5tmr/1
  iac_executive_ctl/9(trig_misc_calcs()) -> [trig_misc_calcs]  "trig_misc_calcs"
  iac_executive_ctl/1(ml_normal_init) -> ml_normal_init/1  "ml_normal_init"
  iac_executive_ctl/7(trig_activate_normal_mode()) -> trig_activate_normal_mode/1  "trig_activate_normal_mode"
  iac_executive_ctl/2(trig_activate_desired_rpm()) -> trig_activate_desired_rpm/1  "trig_activate_desired_rpm"
  iac_executive_ctl/8(trig_fault_code_setting()) -> [trig_fault_code_setting]  "trig_fault_code_setting"
  iac_executive_ctl/6(trig_runup_flag_timer()) -> [trig_runup_flag_timer]  "trig_runup_flag_timer"
  iac_executive_ctl/5(do_failure_mode()) -> [do_failure_mode]  "do_failure_mode"
  iac_executive_ctl/4(trig_crank_mode()) -> [trig_crank_mode]  "trig_crank_mode"
  iac_executive_ctl/3(trig_external_override_mode()) -> [trig_external_override_mode]  "trig_external_override_mode"
  abv_ratio_in/1 -> mode_control/12(abv_ratio_in)
  ratch/1 -> mode_control/11(ratch)
  abv_flowrate_in/1 -> mode_control/10(abv_flowrate_in)
  tcstrt/1 -> mode_control/8(tcstrt)
  [tslpip] -> mode_control/9(tslpip)
  [osc_state] -> mode_control/7(osc_state)
  [osc_ena_0] -> mode_control/6(osc_ena_0)
  [osm_eo_on] -> mode_control/5(osm_eo_on)
  [osm_eo_off] -> mode_control/4(osm_eo_off)
  [trig_crank_mode] -> mode_control/2(trig_crank_mode)
  [do_failure_mode] -> mode_control/3(do_failure_mode)
  mode_control/5(dstpbr) -> dstpbr/1
  [iac_dlt_time] -> fault_code_setting/5(iac_dlt_time)
  abv_percent/1 -> fault_code_setting/2(abv_percent)
  abv_status/1 -> fault_code_setting/3(abv_status)
  [trig_fault_code_setting] -> fault_code_setting/1(trig_fault_code_setting)
  ccm_ena_flg/1 -> fault_code_setting/4(ccm_ena_flg)
  [iac_dlt_time] -> runup_flag_timer/6(iac_dlt_time)
  runup_flag_timer/1(runup_flg) -> runup_flg/1, [runup_flg]
  engine_speed/1 -> runup_flag_timer/5(engine_speed)
  alt_cal_flg/1 -> runup_flag_timer/3(alt_cal_flg)
  dsdrpm/1 -> runup_flag_timer/2(dsdrpm)
  [trig_runup_flag_timer] -> runup_flag_timer/1(trig_runup_flag_timer)
  mode_control/3(hcamfg) -> hcamfg/1
  mode_control/4(iscflg) -> iscflg/1
  mode_control/2(abv_ratio) -> abv_ratio/1
  mode_control/1(abv_flowrate) -> abv_flowrate/1
  [trig_external_override_mode] -> mode_control/1(trig_external_override_mode)
  iac_dlt_time_calc/1(iac_dlt_time) -> [iac_dlt_time], iac_dlt_time/1
  er_isc_hld/1 -> [er_isc_hld], iac_executive_ctl/2(er_isc_hld)
  tfmflg/1 -> [tfmflg], iac_executive_ctl/8(tfmflg)
  osm_eo_on/1 -> [osm_eo_on], iac_executive_ctl/7(osm_eo_on)
  osm_eo_off/1 -> [osm_eo_off], iac_executive_ctl/6(osm_eo_off)
  osc_state/1 -> [osc_state], iac_executive_ctl/5(osc_state)
  osc_ena_0/1 -> [osc_ena_0], iac_executive_ctl/4(osc_ena_0)
  mfmflg/1 -> [mfmflg], iac_executive_ctl/3(mfmflg)
  crkflg/1 -> [crkflg], iac_executive_ctl/1(crkflg)
  iac_executive_ctl/10(do_iac_dlt_time_calc()) -> iac_dlt_time_calc/Trigger  "do_iac_dlt_time_calc"
  [runup_flg] -> iac_executive_ctl/9(runup_flg)
  trig_iac_executive/1 -> iac_executive_ctl/Trigger
  fault_code_setting/1(p1504) -> p1504/1
  runup_flag_timer/2(runuptmr) -> runuptmr/1

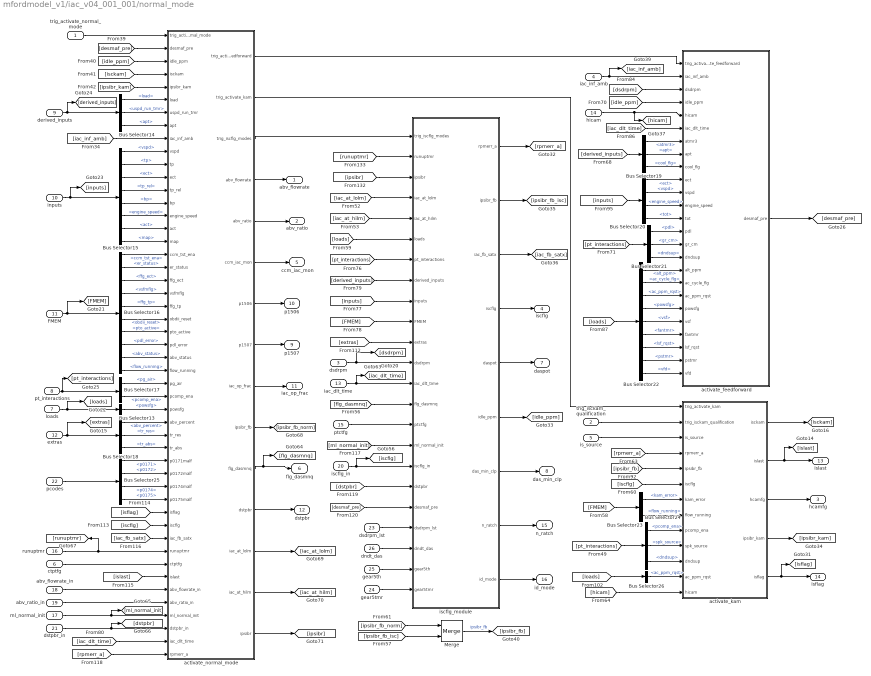
== system mfordmodel_v1/iac_v04_001_001/normal_mode ==
  trig_activate_normal_mode : Inport
  trig_isckam_qualification : Inport  Port=2
  dsdrpm : Inport  Port=3
  iac_inf_amb : Inport  Port=4
  is_source : Inport  Port=5
  ctptfg : Inport  Port=6
  loads : Inport  Port=7
  pt_interactions : Inport  Port=8
  derived_inputs : Inport  Port=9
  inputs : Inport  Port=10
  FMEM : Inport  Port=11
  extras : Inport  Port=12
  iac_dlt_time : Inport  Port=13
  hicam : Inport  Port=14
  ptctfg : Inport  Port=15
  runuptmr : Inport  Port=16
  ml_normal_init : Inport  Port=17
  abv_flowrate_in : Inport  Port=18
  abv_ratio_in : Inport  Port=19
  iscflg_in : Inport  Port=20
  dstpbr_in : Inport  Port=21
  pcodes : Inport  Port=22
  dsdrpm_lst : Inport  Port=23
  gear5tmr : Inport  Port=24
  gear5th : Inport  Port=25
  dndt_das : Inport  Port=26
  Bus Selector13 : BusSelector  OutputSignals=powsfg
  Bus Selector14 : BusSelector  OutputSignals=load,uspd_run_tmr,apt
  Bus Selector15 : BusSelector  OutputSignals=vspd,tp,ect,tp_rel,bp,engine_speed,act,map
  Bus Selector16 : BusSelector  OutputSignals=ccm_tst_ena,er_status,ffg_ect,vsfmflg,ffg_tp,obdii_reset,pto_active,pdl_error,abv_status,flow_running
  Bus Selector17 : BusSelector  OutputSignals=pg_air,pcomp_ena
  Bus Selector18 : BusSelector  OutputSignals=abv_percent,tr_res,tr_abs
  Bus Selector19 : BusSelector  OutputSignals=atmr3,apt,cool_flg
  Bus Selector20 : BusSelector  OutputSignals=ect,vspd,engine_speed,tot
  Bus Selector21 : BusSelector  OutputSignals=pdl,gr_cm,dndsup
  Bus Selector22 : BusSelector  OutputSignals=alt_ppm,ac_cycle_flg,ac_ppm_rqst,powsfg,vsf,fantmr,lsf_rqst,pstmr,vfd
  Bus Selector23 : BusSelector  OutputSignals=kam_error,flow_running
  Bus Selector24 : BusSelector  OutputSignals=pcomp_ena,spk_source,dndsup
  Bus Selector25 : BusSelector  OutputSignals=p0171,p0172,p0174,p0175
  Bus Selector26 : BusSelector  OutputSignals=ac_ppm_rqst
  Merge : Merge
  activate_feedforward : Subsystem
  activate_kam : Subsystem
  activate_normal_mode : Subsystem
  iscflg_module : Subsystem
  abv_flowrate : Outport
  abv_ratio : Outport  Port=2
  hcamfg : Outport  Port=3
  iscflg : Outport  Port=4
  ccm_iac_mon : Outport  Port=5
  flg_dasmnq : Outport  Port=6
  daspot : Outport  Port=7
  das_min_clp : Outport  Port=8
  p1507 : Outport  Port=9
  p1506 : Outport  Port=10
  iac_op_frac : Outport  Port=11
  dstpbr : Outport  Port=12
  islast : Outport  Port=13
  isflag : Outport  Port=14
  n_ratch : Outport  Port=15
  id_mode : Outport  Port=16
  wires:
  iscflg_module/9(id_mode) -> id_mode/1
  iscflg_module/8(n_ratch) -> n_ratch/1
  activate_normal_mode/5(abv_ratio) -> abv_ratio/1
  activate_normal_mode/6(ccm_iac_mon) -> ccm_iac_mon/1
  activate_normal_mode/12(dstpbr) -> dstpbr/1
  activate_normal_mode/13(iac_at_lolm) -> [iac_at_lolm]
  activate_normal_mode/14(iac_at_hilm) -> [iac_at_hilm]
  activate_normal_mode/15(ipsibr) -> [ipsibr]
  FMEM/1 -> Bus Selector16/1, [FMEM]
  Bus Selector17/2 -> activate_normal_mode/29(pcomp_ena)  "<pcomp_ena>"
  loads/1 -> [loads], Bus Selector13/1
  Bus Selector17/1 -> activate_normal_mode/28(pg_air)  "<pg_air>"
  Bus Selector13/1 -> activate_normal_mode/30(powsfg)  "<powsfg>"
  pt_interactions/1 -> Bus Selector17/1, [pt_interactions]
  Bus Selector18/3 -> activate_normal_mode/33(tr_abs)  "<tr_abs>"
  extras/1 -> Bus Selector18/1, [extras]
  Bus Selector18/1 -> activate_normal_mode/31(abv_percent)  "<abv_percent>"
  Bus Selector18/2 -> activate_normal_mode/32(tr_res)  "<tr_res>"
  Bus Selector25/1 -> activate_normal_mode/34(p0171malf)  "<p0171>"
  pcodes/1 -> Bus Selector25/1
  Bus Selector25/2 -> activate_normal_mode/35(p0172malf)  "<p0172>"
  Bus Selector25/3 -> activate_normal_mode/36(p0174malf)  "<p0174>"
  Bus Selector25/4 -> activate_normal_mode/37(p0175malf)  "<p0175>"
  ctptfg/1 -> activate_normal_mode/42(ctptfg)
  abv_flowrate_in/1 -> activate_normal_mode/44(abv_flowrate_in)
  ml_normal_init/1 -> activate_normal_mode/46(ml_normal_init), [ml_normal_init]
  abv_ratio_in/1 -> activate_normal_mode/45(abv_ratio_in)
  dstpbr_in/1 -> activate_normal_mode/47(dstpbr_in), [dstpbr]
  runuptmr/1 -> activate_normal_mode/41(runuptmr), [runuptmr]
  [iac_dlt_time] -> activate_normal_mode/48(iac_dlt_time)
  [rpmerr_a] -> activate_normal_mode/49(rpmerr_a)
  Bus Selector16/10 -> activate_normal_mode/27(flow_running)  "<flow_running>"
  Bus Selector14/1 -> activate_normal_mode/6(load)  "<load>"
  Bus Selector14/2 -> activate_normal_mode/7(uspd_run_tmr)  "<uspd_run_tmr>"
  Bus Selector14/3 -> activate_normal_mode/8(apt)  "<apt>"
  derived_inputs/1 -> Bus Selector14/1, [derived_inputs]
  Bus Selector15/1 -> activate_normal_mode/10(vspd)  "<vspd>"
  Bus Selector15/8 -> activate_normal_mode/17(map)  "<map>"
  Bus Selector15/7 -> activate_normal_mode/16(act)  "<act>"
  Bus Selector15/6 -> activate_normal_mode/15(engine_speed)  "<engine_speed>"
  Bus Selector15/5 -> activate_normal_mode/14(bp)  "<bp>"
  Bus Selector15/4 -> activate_normal_mode/13(tp_rel)  "<tp_rel>"
  Bus Selector15/3 -> activate_normal_mode/12(ect)  "<ect>"
  Bus Selector15/2 -> activate_normal_mode/11(tp)  "<tp>"
  inputs/1 -> Bus Selector15/1, [inputs]
  Bus Selector16/9 -> activate_normal_mode/26(abv_status)  "<abv_status>"
  Bus Selector16/8 -> activate_normal_mode/25(pdl_error)  "<pdl_error>"
  Bus Selector16/7 -> activate_normal_mode/24(pto_active)  "<pto_active>"
  Bus Selector16/6 -> activate_normal_mode/23(obdii_reset)  "<obdii_reset>"
  Bus Selector16/5 -> activate_normal_mode/22(ffg_tp)  "<ffg_tp>"
  Bus Selector16/4 -> activate_normal_mode/21(vsfmflg)  "<vsfmflg>"
  Bus Selector16/3 -> activate_normal_mode/20(ffg_ect)  "<ffg_ect>"
  Bus Selector16/2 -> activate_normal_mode/19(er_status)  "<er_status>"
  Bus Selector16/1 -> activate_normal_mode/18(ccm_tst_ena)  "<ccm_tst_ena>"
  trig_activate_normal_mode/1 -> activate_normal_mode/1(trig_activate_normal_mode)
  [iac_inf_amb] -> activate_normal_mode/9(iac_inf_amb)
  dsdrpm/1 -> iscflg_module/12(dsdrpm), [dsdrpm]
  iac_dlt_time/1 -> iscflg_module/13(iac_dlt_time), [iac_dlt_time]
  iscflg_in/1 -> iscflg_module/17(iscflg_in), [iscflg]
  [desmaf_pre] -> iscflg_module/19(desmaf_pre)
  [iac_at_hilm] -> iscflg_module/5(iac_at_hilm)
  [extras] -> iscflg_module/11(extras)
  [loads] -> iscflg_module/6(loads)
  ptctfg/1 -> iscflg_module/15(ptctfg)
  [dstpbr] -> iscflg_module/18(dstpbr)
  gear5th/1 -> iscflg_module/22(gear5th)
  gear5tmr/1 -> iscflg_module/23(gear5tmr)
  dsdrpm_lst/1 -> iscflg_module/20(dsdrpm_lst)
  [runuptmr] -> iscflg_module/2(runuptmr)
  [ipsibr] -> iscflg_module/3(ipsibr)
  [iac_at_lolm] -> iscflg_module/4(iac_at_lolm)
  [pt_interactions] -> iscflg_module/7(pt_interactions)
  [derived_inputs] -> iscflg_module/8(derived_inputs)
  [FMEM] -> iscflg_module/10(FMEM)
  [inputs] -> iscflg_module/9(inputs)
  [flg_dasmnq] -> iscflg_module/14(flg_dasmnq)
  [ml_normal_init] -> iscflg_module/16(ml_normal_init)
  iscflg_module/3(iac_fb_satx) -> [iac_fb_satx]
  iscflg_module/1(rpmerr_a) -> [rpmerr_a]
  iscflg_module/2(ipsibr_fb) -> [ipsibr_fb_isc]
  iscflg_module/6(idle_ppm) -> [idle_ppm]
  iscflg_module/5(daspot) -> daspot/1
  iscflg_module/4(iscflg) -> iscflg/1
  iscflg_module/7(das_min_clp) -> das_min_clp/1
  dndt_das/1 -> iscflg_module/21(dndt_das)
  activate_normal_mode/3(trig_iscflg_modes) -> iscflg_module/1(trig_iscflg_modes)
  Merge/1 -> [ipsibr_fb]  "ipsibr_fb"
  [ipsibr_fb_isc] -> Merge/2
  [ipsibr_fb_norm] -> Merge/1
  activate_normal_mode/2(trig_activate_kam) -> activate_kam/1(trig_activate_kam)
  hicam/1 -> [hicam], activate_feedforward/5(hicam)
  iac_inf_amb/1 -> activate_feedforward/2(iac_inf_amb), [iac_inf_amb]
  Bus Selector19/1 -> activate_feedforward/7(atmr3)  "<atmr3>"
  [derived_inputs] -> Bus Selector19/1
  Bus Selector19/2 -> activate_feedforward/8(apt)  "<apt>"
  Bus Selector19/3 -> activate_feedforward/9(cool_flg)  "<cool_flg>"
  [inputs] -> Bus Selector20/1
  Bus Selector20/1 -> activate_feedforward/10(ect)  "<ect>"
  Bus Selector20/2 -> activate_feedforward/11(vspd)  "<vspd>"
  Bus Selector20/3 -> activate_feedforward/12(engine_speed)  "<engine_speed>"
  Bus Selector20/4 -> activate_feedforward/13(tot)  "<tot>"
  [pt_interactions] -> Bus Selector21/1
  Bus Selector21/1 -> activate_feedforward/14(pdl)  "<pdl>"
  Bus Selector21/2 -> activate_feedforward/15(gr_cm)  "<gr_cm>"
  Bus Selector21/3 -> activate_feedforward/16(dndsup)  "<dndsup>"
  Bus Selector22/7 -> activate_feedforward/23(lsf_rqst)  "<lsf_rqst>"
  Bus Selector22/6 -> activate_feedforward/22(fantmr)  "<fantmr>"
  Bus Selector22/5 -> activate_feedforward/21(vsf)  "<vsf>"
  [loads] -> Bus Selector22/1
  Bus Selector22/1 -> activate_feedforward/17(alt_ppm)  "<alt_ppm>"
  Bus Selector22/2 -> activate_feedforward/18(ac_cycle_flg)  "<ac_cycle_flg>"
  Bus Selector22/3 -> activate_feedforward/19(ac_ppm_rqst)  "<ac_ppm_rqst>"
  Bus Selector22/4 -> activate_feedforward/20(powsfg)  "<powsfg>"
  [idle_ppm] -> activate_feedforward/4(idle_ppm)
  [dsdrpm] -> activate_feedforward/3(dsdrpm)
  [iac_dlt_time] -> activate_feedforward/6(iac_dlt_time)
  activate_feedforward/1(desmaf_pre) -> [desmaf_pre]
  Bus Selector22/9 -> activate_feedforward/25(vfd)  "<vfd>"
  Bus Selector22/8 -> activate_feedforward/24(pstmr)  "<pstmr>"
  activate_kam/1(isckam) -> [isckam]
  activate_kam/4(ipsibr_kam) -> [ipsibr_kam]
  activate_kam/3(hcamfg) -> hcamfg/1
  [iscflg] -> activate_kam/6(iscflg)
  [rpmerr_a] -> activate_kam/4(rpmerr_a)
  is_source/1 -> activate_kam/3(is_source)
  [ipsibr_fb] -> activate_kam/5(ipsibr_fb)
  Bus Selector23/1 -> activate_kam/7(kam_error)  "<kam_error>"
  Bus Selector23/2 -> activate_kam/8(flow_running)  "<flow_running>"
  Bus Selector24/1 -> activate_kam/9(pcomp_ena)  "<pcomp_ena>"
  Bus Selector24/2 -> activate_kam/10(spk_source)  "<spk_source>"
  Bus Selector24/3 -> activate_kam/11(dndsup)  "<dndsup>"
  [FMEM] -> Bus Selector23/1
  [pt_interactions] -> Bus Selector24/1
  [hicam] -> activate_kam/13(hicam)
  trig_isckam_qualification/1 -> activate_kam/2(trig_isckam_qualification)
  Bus Selector26/1 -> activate_kam/12(ac_ppm_rqst)  "<ac_ppm_rqst>"
  [loads] -> Bus Selector26/1
  activate_kam/2(islast) -> [islast], islast/1
  activate_kam/5(isflag) -> [isflag], isflag/1
  activate_normal_mode/4(abv_flowrate) -> abv_flowrate/1
  activate_normal_mode/8(p1507) -> p1507/1
  activate_normal_mode/7(p1506) -> p1506/1
  activate_normal_mode/9(iac_op_frac) -> iac_op_frac/1
  activate_normal_mode/1(trig_activate_feedforward) -> activate_feedforward/1(trig_activate_feedforward)
  activate_normal_mode/11(flg_dasmnq) -> flg_dasmnq/1, [flg_dasmnq]
  activate_normal_mode/10(ipsibr_fb) -> [ipsibr_fb_norm]
  [desmaf_pre] -> activate_normal_mode/2(desmaf_pre)
  [idle_ppm] -> activate_normal_mode/3(idle_ppm)
  [isckam] -> activate_normal_mode/4(isckam)
  [ipsibr_kam] -> activate_normal_mode/5(ipsibr_kam)
  [iscflg] -> activate_normal_mode/39(iscflg)
  [isflag] -> activate_normal_mode/38(isflag)
  [islast] -> activate_normal_mode/43(islast)
  [iac_fb_satx] -> activate_normal_mode/40(iac_fb_satx)
